simulink model "master_passivity_Hinf_sys"  (R2015a)
settings: Solver=ode45  SolverMode=SingleTasking  StartTime=0.0  StopTime=10.0  RelTol=1e-3
values from neighbouring files (symbols this model uses):
  A = [0 1; 0 -Bm/Mm]    [master_passivity_Hinf.m]
  B = [0; 1/Mm]    [master_passivity_Hinf.m]
  C = [1 0; 0 1]    [master_passivity_Hinf.m]
  D = [0; 0]    [master_passivity_Hinf.m]
  K = M_s * Q_s'    [master_passivity_Hinf.m]
settings Model: Creator=enrico-giordano  LastModifiedBy=enrico-giordano
settings OptimizationCC: BlockReduction=off  BooleanDataType=off
settings DebuggingCC: SaveWithParameterizedLinksMsg=none  UnderspecifiedInitializationDetection=Classic  MergeDetectMultiDrivingBlocksExec=none  SignalResolutionControl=TryResolveAllWithWarning
settings HardwareCC: TargetUnknown=on

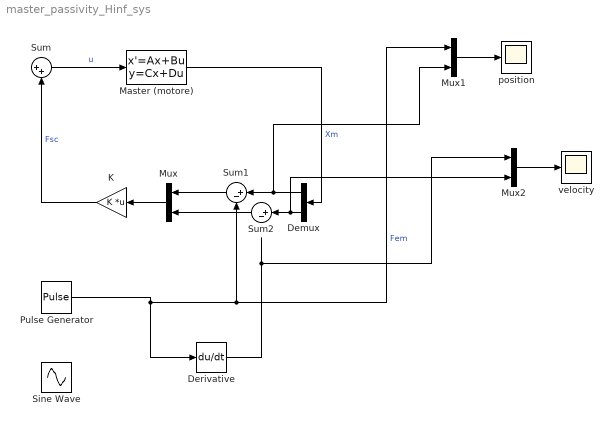
== system master_passivity_Hinf_sys ==
  Demux : Demux  Outputs=2
  Derivative : Derivative
  K : Gain  Gain=K  Multiplication=Matrix(K*u)
  Master (motore) : StateSpace  A=A  B=B  C=C  D=D  X0=0
  Mux : Mux  Inputs=2
  Mux1 : Mux  Inputs=2
  Mux2 : Mux  Inputs=2
  Pulse Generator : DiscretePulseGenerator  PulseType=Time based  PulseWidth=50
  Sine Wave : Sin  Amplitude=10  SampleTime=0
  Sum : Sum  Inputs=|++
  Sum1 : Sum  Inputs=|+-
  Sum2 : Sum  Inputs=|+-
  position : Scope
      settings: TimeRange=10  YMin=-0.6000000000000001  YMax=0.2
  velocity : Scope
      settings: TimeRange=10  YMin=-0.6000000000000001  YMax=0.2
  wires:
  Sum/1 -> Master (motore)/1  "u"
  Master (motore)/1 -> Demux/1  "Xm"
  K/1 -> Sum/2  "Fsc"
  Mux/1 -> K/1
  Demux/1 -> Mux1/2, Sum1/1
  Sum1/1 -> Mux/1
  Pulse Generator/1 -> Derivative/1, Sum1/2, Mux1/1  "Fem"
  Demux/2 -> Mux2/2, Sum2/1
  Mux1/1 -> position/1
  Sum2/1 -> Mux/2
  Derivative/1 -> Mux2/1
  Mux2/1 -> velocity/1
